simulink model "das3implicit_test"  (R2020a)
settings: Solver=FixedStepDiscrete  StartTime=0.0  StopTime=3.999  FixedStep=0.003  RelTol=1e-3  EnableMultiTasking=on
libraries: simulink x2
settings Model: Creator=Dimitra  LastModifiedBy=6000452
settings DataIOCC: LimitDataPoints=on  SaveFormat=Array  SignalLoggingSaveFormat=ModelDataLogs  SaveOutput=off  SignalLogging=off  SaveTime=off  ReturnWorkspaceOutputs=off
settings OptimizationCC: ExpressionDepthLimit=2147483647  LifeSpan=inf
settings DebuggingCC: UnderspecifiedInitializationDetection=Classic  MergeDetectMultiDrivingBlocksExec=none  SolverPrmCheckMsg=warning  FcnCallInpInsideContextMsg=warning  StateNameClashWarn=warning  SFUnexpectedBacktrackingDiag=warning  SFNoUnconditionalDefaultTransitionDiag=warning  SFExecutionAtInitializationDiag=none  ArithmeticOperatorsInVariantConditions=warning
settings HardwareCC: ProdBitPerPointer=32  ProdBitPerSizeT=32  ProdBitPerPtrDiffT=32  ProdLargestAtomicFloat=None  ProdIntDivRoundTo=Undefined  ProdEndianess=Unspecified  ProdWordSize=32  ProdHWDeviceType=32-bit Generic
settings ModelReferenceCC: PropagateSignalLabelsOutOfModel=off
settings SFSimCC: SimUseLocalCustomCode=off  SimParseCustomCode=off  CustomCodeUndefinedFunction=UseInterfaceOnly
settings RTWCC: RTWUseLocalCustomCode=off
settings CodeAppCC: StateflowObjectComments=on
settings GRTTargetCC: TargetLangStandard=C89/C90 (ANSI)  CombineOutputUpdateFcns=off  GRTInterface=on
settings ConfigComp: CovMetricSettings=dw  CovHtmlReporting=on  CovSaveCumulativeToWorkspaceVar=on  CovSaveSingleToWorkspaceVar=on  CovExternalEMLEnable=off

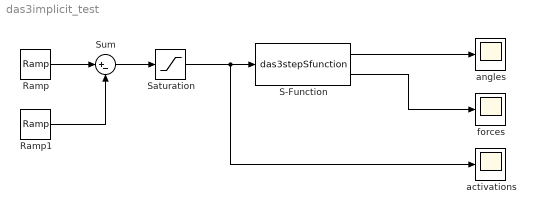
== system das3implicit_test ==
  Ramp : simulink/Sources/Ramp  slope=5  start=0  InitialOutput=zeros(138,1)
  Ramp1 : simulink/Sources/Ramp  slope=10000  start=2  InitialOutput=zeros(138,1)
  S-Function : S-Function  FunctionName=das3stepSfunction  SFunctionDeploymentMode=off  EnableBusSupport=off  SFcnStateName=x
      settings: SFcnIsStateOwnerBlock=on
  Saturation : Saturate  UpperLimit=1  LowerLimit=0
  Sum : Sum  Inputs=|+-
  activations : Scope
  angles : Scope
  forces : Scope
  wires:
  Ramp/1 -> Sum/1
  Ramp1/1 -> Sum/2
  S-Function/1 -> angles/1
  S-Function/2 -> forces/1
  Saturation/1 -> activations/1, S-Function/1
  Sum/1 -> Saturation/1
